simulink model "planar_vtol_sim_HW_04"  (R2018a)
settings: Solver=ode45  StartTime=0.0  StopTime=20  MaxStep=1  MinStep=.75  RelTol=1e-3
InitFcn:
  | planar_vtol_param
undefined symbols (not defined in the file or in its folder): planar_vtol_animation
settings Model: Creator=canla  LastModifiedBy=canla
settings OptimizationCC: LifeSpan=inf

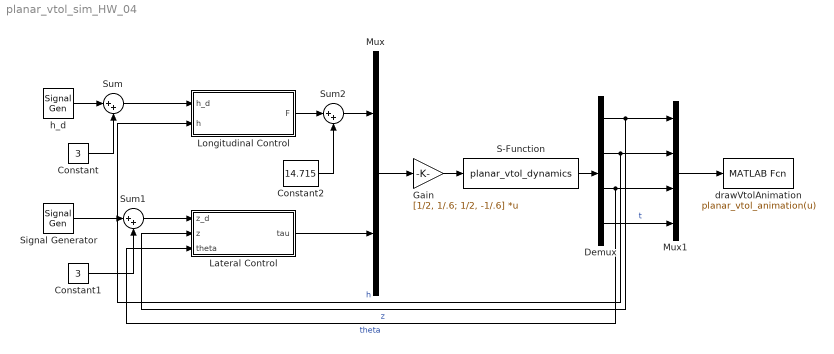
== system planar_vtol_sim_HW_04 ==
  Constant : Constant  Value=3
  Constant1 : Constant  Value=3
  Constant2 : Constant  Value=14.715
  Demux : Demux
  Gain : Gain  Gain=[1/2, 1/.6; 1/2, -1/.6]  Multiplication=Matrix(K*u)
  Lateral Control : Subsystem
  Longitudinal Control : Subsystem
  Mux : Mux  Inputs=2
  Mux1 : Mux
  S-Function : S-Function  FunctionName=planar_vtol_dynamics  Parameters=Pa  SFunctionDeploymentMode=off  EnableBusSupport=off
  Signal Generator : SignalGenerator  WaveForm=square  Amplitude=2.5  Frequency=0.08
  Sum : Sum  Inputs=|++
  Sum1 : Sum  Inputs=|++
  Sum2 : Sum  Inputs=|++
  drawVtolAnimation : MATLABFcn  MATLABFcn=planar_vtol_animation(u)  OutputDimensions=0
  h_d : SignalGenerator  WaveForm=square  Amplitude=2.5  Frequency=0.08
  wires:
  Sum/1 -> Longitudinal Control/1(h_d)
  h_d/1 -> Sum/1
  Constant/1 -> Sum/2
  Signal Generator/1 -> Sum1/1
  Sum1/1 -> Lateral Control/1(z_d)
  Constant1/1 -> Sum1/2
  Lateral Control/1(tau) -> Mux/2
  Longitudinal Control/1(F) -> Sum2/1
  Sum2/1 -> Mux/1
  Constant2/1 -> Sum2/2
  Mux/1 -> Gain/1
  Gain/1 -> S-Function/1
  S-Function/1 -> Demux/1
  Demux/1 -> Mux1/1, Lateral Control/2(z)  "z"
  Demux/2 -> Mux1/2, Longitudinal Control/2(h)  "h"
  Demux/3 -> Mux1/3, Lateral Control/3(theta)  "theta"
  Demux/4 -> Mux1/4  "t"
  Mux1/1 -> drawVtolAnimation/1

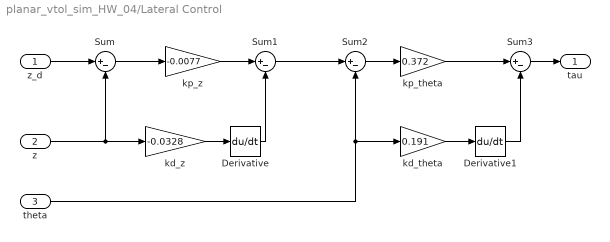
== system planar_vtol_sim_HW_04/Lateral Control ==
  z_d : Inport
  z : Inport  Port=2
  theta : Inport  Port=3
  Derivative : Derivative
  Derivative1 : Derivative
  Sum{,1..3} (4 alike) : Sum  Inputs=|+-
  kd_theta : Gain  Gain=0.191
  kd_z : Gain  Gain=-0.0328
  kp_theta : Gain  Gain=0.372
  kp_z : Gain  Gain=-0.0077
  tau : Outport
  wires:
  z_d/1 -> Sum/1
  Sum/1 -> kp_z/1
  kp_z/1 -> Sum1/1
  Sum1/1 -> Sum2/1
  Sum2/1 -> kp_theta/1
  kp_theta/1 -> Sum3/1
  Sum3/1 -> tau/1
  z/1 -> kd_z/1, Sum/2
  kd_z/1 -> Derivative/1
  Derivative/1 -> Sum1/2
  Derivative1/1 -> Sum3/2
  kd_theta/1 -> Derivative1/1
  theta/1 -> kd_theta/1, Sum2/2

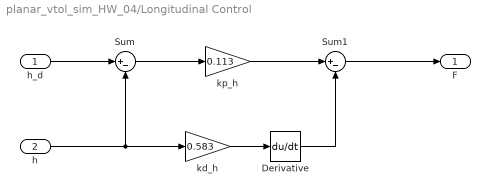
== system planar_vtol_sim_HW_04/Longitudinal Control ==
  h_d : Inport
  h : Inport  Port=2
  Derivative : Derivative
  Sum : Sum  Inputs=|+-
  Sum1 : Sum  Inputs=|+-
  kd_h : Gain  Gain=0.583
  kp_h : Gain  Gain=0.113
  F : Outport
  wires:
  h_d/1 -> Sum/1
  kd_h/1 -> Derivative/1
  Derivative/1 -> Sum1/2
  kp_h/1 -> Sum1/1
  Sum/1 -> kp_h/1
  h/1 -> kd_h/1, Sum/2
  Sum1/1 -> F/1
